simulink model "CinematicaWifi"  (R2025a)
settings: Solver=FixedStepDiscrete  StartTime=0.0  StopTime=inf  FixedStep=0.01  RelTol=1e-3  EnableMultiTasking=on
libraries: arduinowifilib x2, simulink x1
settings Model: SILPILModeSetting=veronly  ExtModeTrigDuration=2  Creator=Antonio  LastModifiedBy=aj
settings SolverCC: AutoInsertRateTranBlk=on
settings OptimizationCC: EnhancedBackFolding=on  PassReuseOutputArgsAs=Individual arguments  ZeroExternalMemoryAtStartup=off  ZeroInternalMemoryAtStartup=off  MaxStackSize=64  OptimizeBlockOrder=speed  DifferentSizesBufferReuse=on  OptimizationCustomize=off  EfficientTunableParamExpr=on
settings DebuggingCC: ParameterTunabilityLossMsg=error
settings HardwareCC: ProdBitPerPointer=32.0  ProdBitPerSizeT=32.0  ProdBitPerPtrDiffT=32.0  ProdLargestAtomicInteger=Long  ProdLargestAtomicFloat=Double  ProdWordSize=32.0  ProdHWDeviceType=ARM Compatible->ARM Cortex
settings SFSimCC: MATLABDynamicMemAlloc=off
settings RTWCC: SystemTargetFile=ert.tlc  HardwareBoard=ESP32-WROOM (Arduino Compatible)  TLCOptions="-aInlineSetEventsForThisBaseRateFcn=TLC_FALSE -aSuppressMultiTaskScheduler=TLC_FALSE  -aRateBasedStepFcn=0"  TemplateMakefile=ert_default_tmf  Toolchain=ESP32  BuildConfiguration=Faster Runs  GPUComputeCapability=3.5  Description=Embedded Coder
settings CodeAppCC: ForceParamTrailComments=on  IgnoreCustomStorageClasses=off  OperatorAnnotations=on  SimulinkDataObjDesc=on  SFDataObjDesc=on  InsertBlockDesc=on
settings ERTTargetCC: ExtModeTransport=3.0  ExtModeAutomaticAllocSize=off  ExtModeStaticAllocSize=65536.0  InlinedParameterPlacement=Hierarchical  DynamicArrayContainerType=coder::array  SupportContinuousTime=on  SupportVariableSizeSignals=on

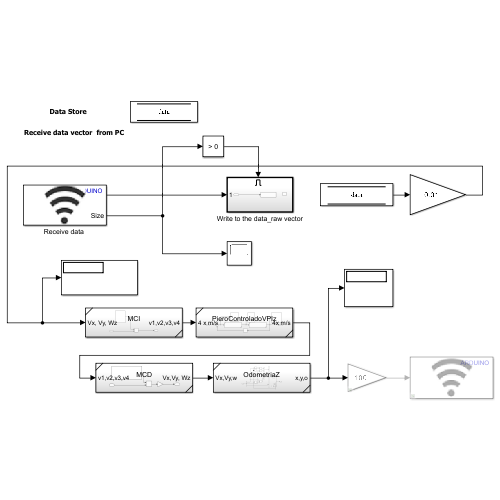
[thumbnail: Simulink's stored preview of the top-level diagram]
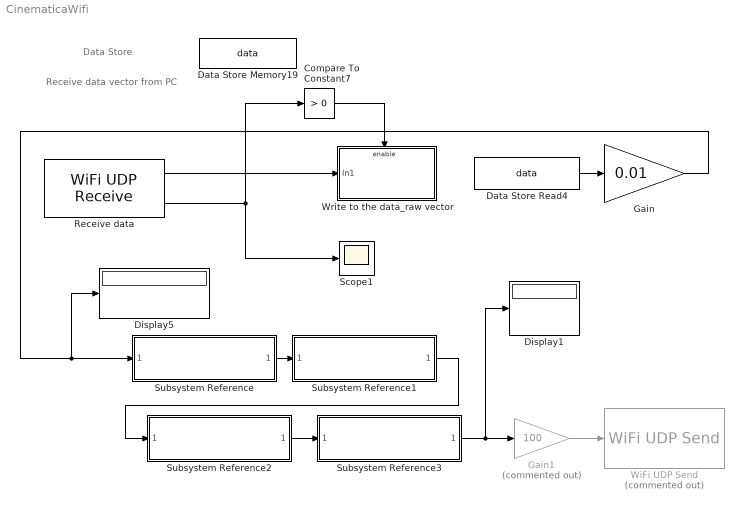
== system CinematicaWifi ==
  note: Receive data vector from PC
  note: Data Store
  Compare To Constant7 : simulink/Logic and Bit Operations/Compare To Constant  relop=>  const=0  OutDataTypeStr=boolean
  Data Store Memory19 : DataStoreMemory  DataStoreName=data  WriteAfterWriteMsg=warning  ShowAdditionalParam=off  OutDataTypeStr=int16  Dimensions=3
  Data Store Read4 : DataStoreRead  DataStoreName=data  IndexOptions=Index vector (dialog)  Indices=1  OutputSizes=1
  Display1 : Display
  Display5 : Display
  Gain : Gain  Gain=0.01  OutDataTypeStr=double
  Gain1 : Gain  Commented=on  Gain=100  OutDataTypeStr=int16
  "Receive data " : arduinowifilib/WiFi UDP Receive  localport=55001  DataType=int16  DataLength=3  SampleTime_=0.01  wifiUDPIndex=2  blockPlatform=ARDUINO  isARMArch=true
  Scope1 : Scope
      settings: ActiveDisplayYMinimum=-1.125  ActiveDisplayYMaximum=10.125
  Subsystem Reference : Subsystem  ReferencedSubsystem=MCI
  Subsystem Reference1 : Subsystem  ReferencedSubsystem=PieroControladoVPIz
  Subsystem Reference2 : Subsystem  ReferencedSubsystem=MCD
  Subsystem Reference3 : Subsystem  ReferencedSubsystem=OdometriaZ
  WiFi UDP Send : arduinowifilib/WiFi UDP Send  Commented=on  remoteIPOctetString=192.168.137.1  remoteport=55002  localport=55001  remoteipoctet1=192  remoteipoctet2=168  remoteipoctet3=137  remoteipoctet4=1  wifiUDPIndex=0  blockPlatform=ARDUINO  isARMArch=false
  Write to the data_raw vector : Subsystem
  wires:
  Gain1/1 -> WiFi UDP Send/1
  Subsystem Reference1/1 -> Subsystem Reference2/1
  Subsystem Reference2/1 -> Subsystem Reference3/1
  Subsystem Reference/1 -> Subsystem Reference1/1
  Subsystem Reference3/1 -> Gain1/1, Display1/1
  "Receive data "/1 -> Write to the data_raw vector/1(In1)
  Data Store Read4/1 -> Gain/1
  "Receive data "/2 -> Compare To Constant7/1, Scope1/1
  Compare To Constant7/1 -> Write to the data_raw vector/Enable
  Gain/1 -> Subsystem Reference/1, Display5/1

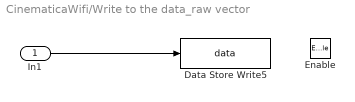
== system CinematicaWifi/Write to the data_raw vector ==
  In1 : Inport
  Enable : EnablePort
  Data Store Write5 : DataStoreWrite  DataStoreName=data  IndexOptions=Index vector (dialog)  Indices=1  OutputSizes=1
  wires:
  In1/1 -> Data Store Write5/1
